simulink model "angleController"  (R2021b)
settings: Solver=VariableStepAuto  StartTime=0.0  StopTime=10  MaxStep=0.02  MinStep=0.01  RelTol=1e-3
undefined symbols (not defined in the file or in its folder): anal_den, anal_num, Ixx
settings Model: Creator=chris  LastModifiedBy=chris

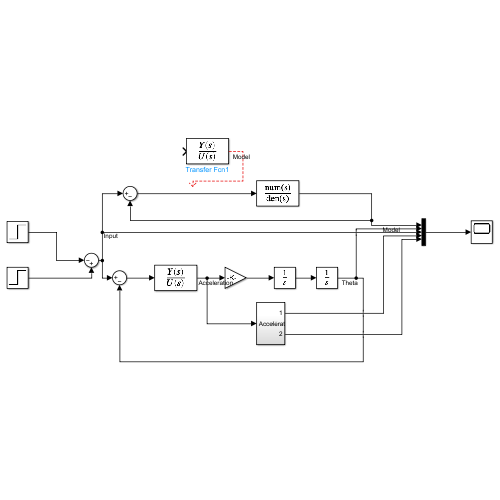
[thumbnail: Simulink's stored preview of the top-level diagram]
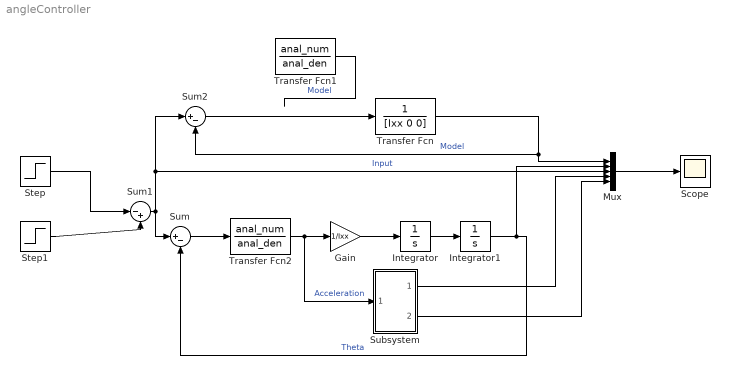
== system angleController ==
  Gain : Gain  Gain=1/Ixx
  Integrator : Integrator
  Integrator1 : Integrator
  Mux : Mux  Inputs=5
  Scope : Scope
  Step : Step  Time=5  SampleTime=0
  Step1 : Step  SampleTime=0
  Subsystem : Subsystem
  Sum : Sum  Inputs=|+-
  Sum1 : Sum  Inputs=|-+
  Sum2 : Sum  Inputs=|+-
  Transfer Fcn : TransferFcn  Denominator=[Ixx 0 0]
  Transfer Fcn1 : TransferFcn  Numerator=anal_num  Denominator=anal_den
  Transfer Fcn2 : TransferFcn  Numerator=anal_num  Denominator=anal_den
  wires:
  Sum/1 -> Transfer Fcn2/1
  Integrator/1 -> Integrator1/1
  Integrator1/1 -> Mux/2, Sum/2  "Theta"
  Mux/1 -> Scope/1
  Step1/1 -> Sum1/2
  Step/1 -> Sum1/1
  Sum1/1 -> Mux/3, Sum2/1, Sum/1  "Input"
  Transfer Fcn/1 -> Sum2/2, Mux/1  "Model"
  Sum2/1 -> Transfer Fcn/1
  Gain/1 -> Integrator/1
  Transfer Fcn1/1 -> ?  "Model"
  Transfer Fcn2/1 -> Subsystem/1(Acceleration), Gain/1  "Acceleration"
  Subsystem/1(Out1) -> Mux/4
  Subsystem/2(Out2) -> Mux/5

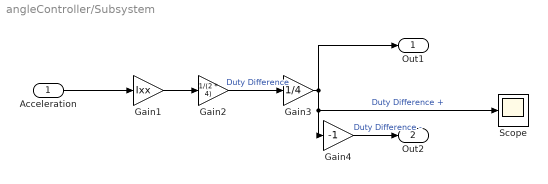
== system angleController/Subsystem ==
  Acceleration : Inport
  Gain1 : Gain  Gain=Ixx
  Gain2 : Gain  Gain=1/(2 * 4)
  Gain3 : Gain  Gain=1/4
  Gain4 : Gain  Gain=-1
  Scope : Scope
  Out1 : Outport
  Out2 : Outport  Port=2
  wires:
  Acceleration/1 -> Gain1/1
  Gain1/1 -> Gain2/1
  Gain2/1 -> Gain3/1  "Duty Difference"
  Gain3/1 -> Scope/1, Gain4/1, Out1/1  "Duty Difference +"
  Gain4/1 -> Out2/1  "Duty Difference -"
